simulink model "ans3"  (R2021a)
settings: Solver=VariableStepAuto  StartTime=0.0  StopTime=10.0  RelTol=1e-3
undefined symbols (not defined in the file): gcbh, xlBlockLoadCallback
libraries: xbsIndex_r4 x853, hdlBasic x20, xrbsMath_r4 x11, xrbsDSP_r4 x10, xrbsImage_r4 x4, xrbsComm_r4 x1
(part 2 of 12)

== system ans3/CIC Filter ==
  note: The CIC filter is constructed out of differentiators and integrators and
      | a sample rate change. This block provides a full precision result and is
      | dynamically built given the parameters entered in the dialog box. The
      | dynamic rebuilding script can switch which side the integrators and
      | differentiators are on and also change between an up and down sampler
      | depending on whether an Interpolator or decimator is selected respectively.
      | The number of stages selected control how many integrators and
      | differentiators are used.
  note: The Interpoiation by 48, 4 stage CIC filter occupies 116 slices.
      | The maximum clock frequency is approximately
      | 308.55 MHz in a Xilinx xc2vp2-7 part (Device speed data version:
      | PRODUCTION 1.121 2005-11-04, ISE 8.1.01i I.25 software, VHDL
      | synthesized with XST).
  In1 : Inport
  Differentiator1 : Subsystem  mask(Differentiator Stage){m=m, output_bitwidth=ceil(stages*log2(rate_change*m) + input_bitwidth), output_binpt=input_binpt}
      mask prompts: m "Differential Delay"; output_bitwidth "Output Bit Width"; output_binpt "Output Binary Point"
      mask help: Multi-Channel Differentiator
      mask init:
      | set_param(gcb, 'LinkStatus', 'none');
  Differentiator2 : Subsystem  mask(Differentiator Stage){m=m, output_bitwidth=ceil(stages*log2(rate_change*m) + input_bitwidth), output_binpt=input_binpt}
      mask prompts: m "Differential Delay"; output_bitwidth "Output Bit Width"; output_binpt "Output Binary Point"
      mask help: Multi-Channel Differentiator
      mask init:
      | set_param(gcb, 'LinkStatus', 'none');
  Differentiator3 : Subsystem  mask(Differentiator Stage){m=m, output_bitwidth=ceil(stages*log2(rate_change*m) + input_bitwidth), output_binpt=input_binpt}
      mask prompts: m "Differential Delay"; output_bitwidth "Output Bit Width"; output_binpt "Output Binary Point"
      mask help: Multi-Channel Differentiator
      mask init:
      | set_param(gcb, 'LinkStatus', 'none');
  Down Sample : hdlBasic/Down Sample  sample_ratio=rate_change  sample_phase=First Value of Frame  en=off  rst=off  latency=1  XmcBlockStatus=1  maskContainerNames=group1  block_type=dsamp  block_config=sysgen:Downsample_config
  Integrator1 : Subsystem  mask(Integrator Stage){output_bitwidth=ceil(stages*log2(rate_change*m) + input_bitwidth)}
      mask prompts: output_bitwidth "Output Bit Width"
      mask help: Multi Channel Integrator
      mask init:
      | set_param(gcb, 'LinkStatus', 'none');
      settings: CopyFcn=set_param(gcb, 'LinkStatus', 'none');
  Integrator2 : Subsystem  mask(Integrator Stage){output_bitwidth=ceil(stages*log2(rate_change*m) + input_bitwidth)}
      mask prompts: output_bitwidth "Output Bit Width"
      mask help: Multi Channel Integrator
      mask init:
      | set_param(gcb, 'LinkStatus', 'none');
      settings: CopyFcn=set_param(gcb, 'LinkStatus', 'none');
  Integrator3 : Subsystem  mask(Integrator Stage){output_bitwidth=ceil(stages*log2(rate_change*m) + input_bitwidth)}
      mask prompts: output_bitwidth "Output Bit Width"
      mask help: Multi Channel Integrator
      mask init:
      | set_param(gcb, 'LinkStatus', 'none');
      settings: CopyFcn=set_param(gcb, 'LinkStatus', 'none');
  Out1 : Outport  VectorParamsAs1DForOutWhenUnconnected=off
  wires:
  In1/1 -> Integrator1/1(In1)
  Down Sample/1 -> Differentiator1/1(In1)
  Integrator1/1(Out1) -> Integrator2/1(In1)
  Differentiator1/1(Out1) -> Differentiator2/1(In1)
  Integrator2/1(Out1) -> Integrator3/1(In1)
  Differentiator2/1(Out1) -> Differentiator3/1(In1)
  Integrator3/1(Out1) -> Down Sample/1
  Differentiator3/1(Out1) -> Out1/1

== system ans3/CIC Filter1 ==
  note: The CIC filter is constructed out of differentiators and integrators and
      | a sample rate change. This block provides a full precision result and is
      | dynamically built given the parameters entered in the dialog box. The
      | dynamic rebuilding script can switch which side the integrators and
      | differentiators are on and also change between an up and down sampler
      | depending on whether an Interpolator or decimator is selected respectively.
      | The number of stages selected control how many integrators and
      | differentiators are used.
  note: The Interpoiation by 48, 4 stage CIC filter occupies 116 slices.
      | The maximum clock frequency is approximately
      | 308.55 MHz in a Xilinx xc2vp2-7 part (Device speed data version:
      | PRODUCTION 1.121 2005-11-04, ISE 8.1.01i I.25 software, VHDL
      | synthesized with XST).
  In1 : Inport
  Differentiator1 : Subsystem  mask(Differentiator Stage){m=m, output_bitwidth=ceil(stages*log2(rate_change*m) + input_bitwidth), output_binpt=input_binpt}
      mask prompts: m "Differential Delay"; output_bitwidth "Output Bit Width"; output_binpt "Output Binary Point"
      mask help: Multi-Channel Differentiator
      mask init:
      | set_param(gcb, 'LinkStatus', 'none');
  Differentiator2 : Subsystem  mask(Differentiator Stage){m=m, output_bitwidth=ceil(stages*log2(rate_change*m) + input_bitwidth), output_binpt=input_binpt}
      mask prompts: m "Differential Delay"; output_bitwidth "Output Bit Width"; output_binpt "Output Binary Point"
      mask help: Multi-Channel Differentiator
      mask init:
      | set_param(gcb, 'LinkStatus', 'none');
  Differentiator3 : Subsystem  mask(Differentiator Stage){m=m, output_bitwidth=ceil(stages*log2(rate_change*m) + input_bitwidth), output_binpt=input_binpt}
      mask prompts: m "Differential Delay"; output_bitwidth "Output Bit Width"; output_binpt "Output Binary Point"
      mask help: Multi-Channel Differentiator
      mask init:
      | set_param(gcb, 'LinkStatus', 'none');
  Down Sample : hdlBasic/Down Sample  sample_ratio=rate_change  sample_phase=First Value of Frame  en=off  rst=off  latency=1  XmcBlockStatus=1  maskContainerNames=group1  block_type=dsamp  block_config=sysgen:Downsample_config
  Integrator1 : Subsystem  mask(Integrator Stage){output_bitwidth=ceil(stages*log2(rate_change*m) + input_bitwidth)}
      mask prompts: output_bitwidth "Output Bit Width"
      mask help: Multi Channel Integrator
      mask init:
      | set_param(gcb, 'LinkStatus', 'none');
      settings: CopyFcn=set_param(gcb, 'LinkStatus', 'none');
  Integrator2 : Subsystem  mask(Integrator Stage){output_bitwidth=ceil(stages*log2(rate_change*m) + input_bitwidth)}
      mask prompts: output_bitwidth "Output Bit Width"
      mask help: Multi Channel Integrator
      mask init:
      | set_param(gcb, 'LinkStatus', 'none');
      settings: CopyFcn=set_param(gcb, 'LinkStatus', 'none');
  Integrator3 : Subsystem  mask(Integrator Stage){output_bitwidth=ceil(stages*log2(rate_change*m) + input_bitwidth)}
      mask prompts: output_bitwidth "Output Bit Width"
      mask help: Multi Channel Integrator
      mask init:
      | set_param(gcb, 'LinkStatus', 'none');
      settings: CopyFcn=set_param(gcb, 'LinkStatus', 'none');
  Out1 : Outport  VectorParamsAs1DForOutWhenUnconnected=off
  wires:
  In1/1 -> Integrator1/1(In1)
  Down Sample/1 -> Differentiator1/1(In1)
  Integrator1/1(Out1) -> Integrator2/1(In1)
  Differentiator1/1(Out1) -> Differentiator2/1(In1)
  Integrator2/1(Out1) -> Integrator3/1(In1)
  Differentiator2/1(Out1) -> Differentiator3/1(In1)
  Integrator3/1(Out1) -> Down Sample/1
  Differentiator3/1(Out1) -> Out1/1

== system ans3/CORDIC ATAN ==
  note: The CORDIC algorithm is implemented in 3 steps.
      |
      | Step 1: Coarse Angle Rotation.  The algorithm converges only for angles between -pi/2 and pi/2, so if x < zero, the input vector is reflected
      | to the 1st or 3rd quadrant by making the x-coordinate non-negative.
      |
      | Step 2: Fine Angle Rotation.  For rectangular-to-polar conversion, the resulting vector is rotated through progressively smaller angles, such that y goes
      | to zero. In the i-th stage, the angular rotation is by either +/- atan(1/2^i), depending on whether or not its input y is less than or greater than zero.
      |
      | Step 3: Angle Correction. If there was a reflection applied in Step 1, this step applies the appropriate angle correction by subtracting it from +/- pi.
  x : Inport
  y : Inport  Port=2
  CORDIC Pipe Balance : xbsIndex_r4/Delay  rst=off  infoeditControl=Selection of Reset will increase slice count due to use of real FFs and instead of SRLs  en=off  latency=sum(pipeline)  dbl_ovrd=off  reg_retiming=off  block_type=delay
      settings: infoedit="Delay line having  configurable length.<P><P>Hardware notes: A delay line is a chain, each link of which is an SRL16 followed by a flip-flop. If register retiming is enabled, the delay line is a chain of flip-flops."  xl_area=[0, 0, 0, 0, 0, 0, 0]  block_version=VER_STRING_GOES_HERE
  CORDIC Pipe Balance1 : xbsIndex_r4/Delay  rst=off  infoeditControl=Selection of Reset will increase slice count due to use of real FFs and instead of SRLs  en=off  latency=sum(pipeline)+1  dbl_ovrd=off  reg_retiming=off  block_type=delay
      settings: infoedit="Delay line having  configurable length.<P><P>Hardware notes: A delay line is a chain, each link of which is an SRL16 followed by a flip-flop. If register retiming is enabled, the delay line is a chain of flip-flops."  xl_area=[0, 0, 0, 0, 0, 0, 0]  block_version=VER_STRING_GOES_HERE
  CORDIC Pipe Balance2 : xbsIndex_r4/Delay  rst=off  infoeditControl=Selection of Reset will increase slice count due to use of real FFs and instead of SRLs  en=off  latency=1  dbl_ovrd=off  reg_retiming=off  block_type=delay
      settings: infoedit="Delay line having  configurable length.<P><P>Hardware notes: A delay line is a chain, each link of which is an SRL16 followed by a flip-flop. If register retiming is enabled, the delay line is a chain of flip-flops."  xl_area=[0, 0, 0, 0, 0, 0, 0]  block_version=VER_STRING_GOES_HERE
  CORDIC Fine Angle PE : Subsystem  mask(CORDIC parallel PE){}
      mask init:
      | [bg,fg] = xlcmap('XBlock',0);
      | iPos = get_param(gcb,'Position');
      | iWidth=iPos(3)-iPos(1); iHeight=iPos(4)-iPos(2);
      | iCx=iWidth/2;
      | iCy=iHeight/2;
      | [logoX, logoY] = xlogo(iPos);
      mask Display:
      | patch([0 iWidth iWidth 0],[0 0 iHeight iHeight] , bg);
      | patch(logoX,logoY , fg);
      | port_label('input',1,'x');
      | port_label('input',2,'y');
      | port_label('input',3,'z');
      | port_label('output',1,'X');
      | port_label('output',2,'Z');
      | plot([0 0 iWidth iWidth 0], [0 iHeight iHeight 0 0]);
  Constant : xbsIndex_r4/Constant  const=0  gui_display_data_type=Fixed-point  arith_type=Signed (2's comp)  n_bits=pe_nbits  bin_pt=pe_binpt  preci_type=Single  exp_width=8  frac_width=24  explicit_period=off  period=1  equ=P=C  opselect=C  inp2=PCIN>>17  opr=+  inp1=P  carry=CIN  dbl_ovrd=off  block_type=constant
      settings: block_version=VER_STRING_GOES_HERE
  Quadrant Correct : Subsystem
      mask init:
      | [bg,fg] = xlcmap('XBlock',0);
      | iPos = get_param(gcb,'Position');
      | iWidth=iPos(3)-iPos(1); iHeight=iPos(4)-iPos(2);
      | iCx=iWidth/2;
      | iCy=iHeight/2;
      | [logoX, logoY] = xlogo(iPos);
      mask Display:
      | patch([0 iWidth iWidth 0],[0 0 iHeight iHeight] , bg);
      | patch(logoX,logoY , fg);
      | port_label('input',1,'Z in');
      | port_label('input',2,'sgn(y)');
      | port_label('input',3,'sgn(x)');
      | port_label('output',1,'Z');
      | plot([0 0 iWidth iWidth 0], [0 iHeight iHeight 0 0]);
  Quadrant Map : Subsystem
      mask init:
      | [bg,fg] = xlcmap('XBlock',0);
      | iPos = get_param(gcb,'Position');
      | iWidth=iPos(3)-iPos(1); iHeight=iPos(4)-iPos(2);
      | iCx=iWidth/2;
      | iCy=iHeight/2;
      | [logoX, logoY] = xlogo(iPos);
      mask Display:
      | patch([0 iWidth iWidth 0],[0 0 iHeight iHeight] , bg);
      | patch(logoX,logoY , fg);
      | port_label('input',1,'x');
      | port_label('input',2,'y');
      | port_label('output',1,'X');
      | port_label('output',2,'Y');
      | port_label('output',3,'sgn(y)');
      | port_label('output',4,'sgn(x)');
      | plot([0 0 iWidth iWidth 0], [0 iHeight iHeight 0 0]);
  X : Outport  VectorParamsAs1DForOutWhenUnconnected=off
  Z : Outport  Port=2  VectorParamsAs1DForOutWhenUnconnected=off
  wires:
  Constant/1 -> CORDIC Fine Angle PE/3(z)
  Quadrant Map/1(X) -> CORDIC Fine Angle PE/1(x)
  Quadrant Map/2(Y) -> CORDIC Fine Angle PE/2(y)
  x/1 -> Quadrant Map/1(x)
  y/1 -> Quadrant Map/2(y)
  Quadrant Map/3(sign(y)) -> CORDIC Pipe Balance/1
  Quadrant Map/4(sign(x)) -> CORDIC Pipe Balance1/1
  CORDIC Pipe Balance/1 -> Quadrant Correct/2(PI_ addsub)
  CORDIC Pipe Balance1/1 -> Quadrant Correct/3(Z MUX SEL)
  CORDIC Fine Angle PE/2(Z) -> Quadrant Correct/1(Z IN)
  Quadrant Correct/1(Z) -> Z/1
  CORDIC Fine Angle PE/1(X) -> CORDIC Pipe Balance2/1
  CORDIC Pipe Balance2/1 -> X/1

== system ans3/CORDIC DIVIDER ==
  note: The CORDIC Divider algorithm is implemented in 4 steps.
      |
      | Step 1: Co-ordinate Rotation.  The CORDIC algorithm converges only for positive values of x, so if x < zero, the input vector is
      | reflected to the 1st or 3rd quadrant by making the x-coordinate non-negative. For normalizing X and Y, Y is always mapped to
      | a non-negative value. The Divider circuit has been designed to converge for all values of X and Y, except for the most negative value .
      |
      | Step 2: Normalization.  The CORDIC algorithm converges only for y <= 2 x. For  x > y, both the inputs X and Y are shifted to the
      | left till they have a 1 in the most significant bit (MSB).  The relative shift of Y over X is recorded and passed on to the Quadrant
      | Correct Stage.
      |
      | Step 3: Linear Rotations.  For ratio calculation, the resulting vector is rotated through progressively smaller angles, such that y goes
      | to zero. In the i-th stage, the rotation yields +/- y/x, depending on whether the input y is less than or greater than zero.
      |
      | Step 4: Co-ordinate Correction. If the axis was rotated Step 1 and a relative shift was applied to Y over X, this step assigns the appropriate
      | sign to the resulting ratio and multiplies it with 2^(relative_shift of Y over X).
  x : Inport
  y : Inport  Port=2
  Constant2 : xbsIndex_r4/Constant  const=0  gui_display_data_type=Fixed-point  arith_type=Signed (2's comp)  n_bits=stages+2  bin_pt=stages  preci_type=Single  exp_width=8  frac_width=24  explicit_period=off  period=1  equ=P=C  opselect=C  inp2=PCIN>>17  opr=+  inp1=P  carry=CIN  dbl_ovrd=off  block_type=constant
      settings: block_version=VER_STRING_GOES_HERE
  Delay : xbsIndex_r4/Delay  rst=off  infoeditControl=Selection of Reset will increase slice count due to use of real FFs and instead of SRLs  en=off  latency=sum(pipeline)  dbl_ovrd=off  reg_retiming=off  block_type=delay
      settings: infoedit="Delay line having  configurable length.<P><P>Hardware notes: A delay line is a chain, each link of which is an SRL16 followed by a flip-flop. If register retiming is enabled, the delay line is a chain of flip-flops."  xl_area=[1 1 0 1 0 0 0]  block_version=VER_STRING_GOES_HERE
  Delay1 : xbsIndex_r4/Delay  rst=off  infoeditControl=Selection of Reset will increase slice count due to use of real FFs and instead of SRLs  en=off  latency=sum(pipeline)  dbl_ovrd=off  reg_retiming=off  block_type=delay
      settings: infoedit="Delay line having  configurable length.<P><P>Hardware notes: A delay line is a chain, each link of which is an SRL16 followed by a flip-flop. If register retiming is enabled, the delay line is a chain of flip-flops."  xl_area=[2 4 0 4 0 0 0]  block_version=VER_STRING_GOES_HERE
  Iterative Divider : Subsystem  mask(CORDIC Iterative Divider){}
      mask init:
      | [bg,fg] = xlcmap('XBlock',0);
      | iPos = get_param(gcb,'Position');
      | iWidth=iPos(3)-iPos(1); iHeight=iPos(4)-iPos(2);
      | iCx=iWidth/2;
      | iCy=iHeight/2;
      | [logoX, logoY] = xlogo(iPos);
      mask Display:
      | patch([0 iWidth iWidth 0],[0 0 iHeight iHeight] , bg);
      | patch(logoX,logoY , fg);
      | port_label('input',1,'x');
      | port_label('input',2,'y');
      | port_label('input',3,'z');
      | port_label('output',1,'Z');
      | plot([0 0 iWidth iWidth 0], [0 iHeight iHeight 0 0]);
  Quadrant Correct : Subsystem  mask{num_width=num_width, num_binpt=num_binpt}
      mask prompts: num_width "Data Width"; num_binpt "Data Binary Point"
      mask init:
      | [bg,fg] = xlcmap('XBlock',0);
      | iPos = get_param(gcb,'Position');
      | iWidth=iPos(3)-iPos(1); iHeight=iPos(4)-iPos(2);
      | iCx=iWidth/2;
      | iCy=iHeight/2;
      | [logoX, logoY] = xlogo(iPos);
      mask Display:
      | patch([0 iWidth iWidth 0],[0 0 iHeight iHeight] , bg);
      | patch(logoX,logoY , fg);
      | port_label('input',1,'z');
      | port_label('input',2,'sign');
      | port_label('input',3,'norm');
      | port_label('output',1,'y/x');
      | plot([0 0 iWidth iWidth 0], [0 iHeight iHeight 0 0]);
  Quadrant Map : Subsystem  mask{num_width=num_width, num_binpt=num_binpt}
      mask prompts: num_binpt "Num_bin_pt"
      mask init:
      | [bg,fg] = xlcmap('XBlock',0);
      | iPos = get_param(gcb,'Position');
      | iWidth=iPos(3)-iPos(1); iHeight=iPos(4)-iPos(2);
      | iCx=iWidth/2;
      | iCy=iHeight/2;
      | [logoX, logoY] = xlogo(iPos);
      mask Display:
      | patch([0 iWidth iWidth 0],[0 0 iHeight iHeight] , bg);
      | patch(logoX,logoY , fg);
      | port_label('input',1,'x');
      | port_label('input',2,'y');
      | port_label('output',1,'norm_x');
      | port_label('output',2,'norm_y');
      | port_label('output',3,'sign');
      | port_label('output',4,'index');
      | plot([0 0 iWidth iWidth 0], [0 iHeight iHeight 0 0]);
  div : Outport  VectorParamsAs1DForOutWhenUnconnected=off
  wires:
  Quadrant Correct/1(Z) -> div/1
  y/1 -> Quadrant Map/2(y)
  x/1 -> Quadrant Map/1(x)
  Delay1/1 -> Quadrant Correct/3(norm)
  Quadrant Map/4(index) -> Delay1/1
  Delay/1 -> Quadrant Correct/2(sign)
  Quadrant Map/3(sign) -> Delay/1
  Iterative Divider/1(Z) -> Quadrant Correct/1(z)
  Quadrant Map/2(norm_Y) -> Iterative Divider/2(y)
  Quadrant Map/1(norm_X) -> Iterative Divider/1(x)
  Constant2/1 -> Iterative Divider/3(z)

== system ans3/CORDIC LOG ==
  note: The CORDIC Natural Log algorithm is implemented in 4 steps.
      |
      | Step 1: Co-ordinate Rotation.  The CORDIC algorithm converges only for positive values of x. If x < zero, the input data is
      | converted to a non-negative number. If x = 0, a zero detect flag is passed along to the output stage. The Log circuit has been
      | designed to converge for all values of X, except for the most negative value .
      |
      | Step 2: Normalization.  The CORDIC algorithm converges only for 0.5 <= x < 1.0. During normalization, the input X is shifted to the
      | left till it has a 1 in the most significant bit.The log output is derived using the identity log( w) = 2*atanh{ (w-l) / (w+1) }.
      | Based on this identity the input w gets mapped to, X = w + 1 and Y = w - 1.
      |
      | Step 3: Hyperbolic Rotations.  For atanh{ (w-l) / (w+1) }. calculation, the resulting vector is rotated through progressively smaller
      | angles, such that y goes to zero.
      |
      | Step 4: Co-ordinate Correction. If the input was negative  a CMPLX_PI flag is porvided at the output for adding PI if a complex output is desired.
      | If a left shift was applied to X, this step adjusts the output by using the equation log (w * 2^E) = log (w) + E * log (2).
  x : Inport
  CORDIC Fine Angle PE : Subsystem  mask(CORDIC parallel PE){stages=stages, pe_nbits=pe_nbits+1, pe_binpt=pe_nbits-1, pipeline_x=pipeline, prev_stages=7, pipeline=[1  1  1  1  1  1  1]}
      mask prompts: stages "Number of Stages"; pe_nbits "Number of Bits"; pe_binpt "Binary Point Position"; pipeline_x "Pipeline Stage Value"; prev_stages "Previous Stages"; pipeline "Previous Pipeline Stage Value"
      mask init:
      | [bg,fg] = xlcmap('XBlock',0);
      | iPos = get_param(gcb,'Position');
      | iWidth=iPos(3)-iPos(1); iHeight=iPos(4)-iPos(2);
      | iCx=iWidth/2;
      | iCy=iHeight/2;
      | [logoX, logoY] = xlogo(iPos);
      | set_param(gcb,'LinkStatus', 'none');
      | sav_gcb=gcb;
      | stages = round(sum(abs(stages)));
      | if (stages == 0)
      | 	stages = prev_stages;
      | end
      | x = zeros(1,stages);
      | pipe_size = max(size(pipeline_x));
      | if pipe_size >= stages
      | 	x(1,1:stages) = pipeline_x(1,1:stages);
      | else
      | 	x(1,1:pipe_size) = pipeline_x(1,1:pipe_size);
      | end
      | 
      | if (stages ~=prev_stages)
      | 	pipeline = x;
      | 	a=find_system(sav_gcb, 'lookUnderMasks', 'all', 'FollowLinks','on','masktype', 'CORDIC iteration PE');
      | 	for i= 2:length(a)
      | 		for j=1:3
      | 		    delete_line(sav_gcb, ['CORDIC PE' int2str(i-1) '/' int2str(j)], ['CORDIC PE' int2str(i) '/' int2str(j)]);
      | 		end
      | 	end
      | 	delete_line(sav_gcb, ['CORDIC PE' int2str(length(a)) '/1'],'T1/1');
      | 	delete_line(sav_gcb, ['CORDIC PE' int2str(length(a)) '/2'],'T2/1');
      | 	delete_line(sav_gcb, ['CORDIC PE' int2str(length(a)) '/3'],'Z/1');
      | 	
      | 	for i=2:length(a)
      |       delete_block(a{i});
      | 	end
      | 	ite_stage=1;
      | 	repeat_stage=4;
      | 	dec_stage=0;
      | 	for i=2:stages
      |         ite_stage= i-dec_stage;
      | 		if(repeat_stage==ite_stage-1)
      |             ite_stage=ite_stage-1;
      | 			repeat_stage=repeat_stage*3+1;
      | 			dec_stage=dec_stage+1;
      | 		end
      |         add_block([sav_gcb '/CORDIC PE1'], [sav_gcb '/CORDIC PE' int2str(i)],'ii',int2str(ite_stage),'pipeline',['pipeline(1,' int2str(i) ')'],'position',[150+(i-1)*125, 70, 205+(i-1)*125, 130]);
      | 	end
      |     set_param([sav_gcb '/' 'T1'], 'Position', [150+stages*125, 73, 180+stages*125, 87]);
      |     set_param([sav_gcb '/' 'T2'], 'Position', [210+stages*125, 92, 225+stages*125, 108]);
      | 	set_param([sav_gcb '/' 'Z'], 'Position', [270+stages*125, 111, 270+stages*125, 129]);
      |     for i= 2:stages
      | 		for j=1:3
      | 		    add_line(sav_gcb, ['CORDIC PE' int2str(i-1) '/' int2str(j)], ['CORDIC PE' int2str(i) '/' int2str(j)]);
      | 		end
      | 	end
      |     add_line(sav_gcb, ['CORDIC PE' int2str(stages) '/1'],'T1/1');
      | 	add_line(sav_gcb, ['CORDIC PE' int2str(stages) '/2'],'T2/1');
      | 	add_line(sav_gcb, ['CORDIC PE' int2str(stages) '/3'],'Z/1');
      | 	find_system(sav_gcb, 'lookUnderMasks', 'all', 'FollowLinks', 'on', 'MaskType','Xilinx Slice Block');
      | 	set_param(sav_gcb, 'prev_stages',int2str(stages));
      | 	set_param(sav_gcb, 'pipeline', [ '[' int2str(x) ']']);
      | end
      | 
      | if (sum(pipeline~=x))
      | 	pipeline = x;
      | 	set_param(sav_gcb, 'pipeline', [ '[' int2str(x) ']']);
      | end
      mask Display:
      | patch([0 iWidth iWidth 0],[0 0 iHeight iHeight] , bg);
      | patch(logoX,logoY , fg);
      | port_label('input',1,'x');
      | port_label('input',2,'y');
      | port_label('input',3,'z');
      | port_label('input',4,'shift');
      | port_label('input',5,'sgn(x)');
      | port_label('input',6,'0_det');
      | port_label('output',1,'Z');
      | port_label('output',2,'shift');
      | port_label('output',3,'sgn(x)');
      | port_label('output',4,'0_det');
      | plot([0 0 iWidth iWidth 0], [0 iHeight iHeight 0 0]);
  Quadrant Correct : Subsystem  mask{pe_nbits=pe_nbits, pe_binpt=pe_binpt, k_val=0, k_bits=0}
      mask prompts: pe_nbits "Number of Bits"; pe_binpt "Binary Point Position"; k_val "Constant Value"; k_bits "Constant Bits"
      mask init:
      | [bg,fg] = xlcmap('XBlock',0);
      | iPos = get_param(gcb,'Position');
      | iWidth=iPos(3)-iPos(1); iHeight=iPos(4)-iPos(2);
      | iCx=iWidth/2;
      | iCy=iHeight/2;
      | [logoX, logoY] = xlogo(iPos);
      | t = pe_nbits-pe_binpt-1;
      | if (t== 0)
      | 	k_val = 0;
      | 	k_bits = 1;
      | else
      | 	k_val= t;
      | 	k_bits = ceil(log2(t+1));
      | end
      mask Display:
      | patch([0 iWidth iWidth 0],[0 0 iHeight iHeight] , bg);
      | patch(logoX,logoY , fg);
      | port_label('input',1,'X');
      | port_label('input',2,'shift');
      | port_label('input',3,'sgn(x)');
      | port_label('input',4,'0_det');
      | port_label('output',1,'log X');
      | port_label('output',2,'CMPLX_PI');
      | plot([0 0 iWidth iWidth 0], [0 iHeight iHeight 0 0]);
  Quadrant Map : Subsystem
      mask init:
      | [bg,fg] = xlcmap('XBlock',0);
      | iPos = get_param(gcb,'Position');
      | iWidth=iPos(3)-iPos(1); iHeight=iPos(4)-iPos(2);
      | iCx=iWidth/2;
      | iCy=iHeight/2;
      | [logoX, logoY] = xlogo(iPos);
      mask Display:
      | patch([0 iWidth iWidth 0],[0 0 iHeight iHeight] , bg);
      | patch(logoX,logoY , fg);
      | port_label('input',1,'x');
      | port_label('output',1,'X');
      | port_label('output',2,'Y');
      | port_label('output',3,'Z');
      | port_label('output',4,'shift');
      | port_label('output',5,'sgn(x)');
      | port_label('output',6,'0_det');
      | plot([0 0 iWidth iWidth 0], [0 iHeight iHeight 0 0]);
  logx : Outport  VectorParamsAs1DForOutWhenUnconnected=off
  CMPLX_PI : Outport  Port=2  VectorParamsAs1DForOutWhenUnconnected=off
  wires:
  CORDIC Fine Angle PE/3(sign_dly) -> Quadrant Correct/3(sign_x)
  CORDIC Fine Angle PE/2(shift_dly) -> Quadrant Correct/2(shift)
  Quadrant Map/5(sign) -> CORDIC Fine Angle PE/5(sign)
  Quadrant Map/6(zero_detect) -> CORDIC Fine Angle PE/6(zero_detect)
  Quadrant Map/4(shift1) -> CORDIC Fine Angle PE/4(shift1)
  Quadrant Map/3(shift) -> CORDIC Fine Angle PE/3(z)
  Quadrant Map/2(Y) -> CORDIC Fine Angle PE/2(y)
  Quadrant Map/1(X) -> CORDIC Fine Angle PE/1(x)
  Quadrant Correct/2(CMPLX_PI) -> CMPLX_PI/1
  CORDIC Fine Angle PE/4(zero_detect_dly) -> Quadrant Correct/4(zero_detect)
  x/1 -> Quadrant Map/1(x)
  CORDIC Fine Angle PE/1(Z) -> Quadrant Correct/1(X)
  Quadrant Correct/1(Z) -> logx/1

== system ans3/CORDIC SINCOS ==
  note: The CORDIC algorithm is implemented in 3 steps.
      |
      | Step 1: Coarse Angle Rotation.  The algorithm converges only for angles between -pi/2 and pi/2. If  z > pi/2, the input angle is reflected
      |  to the 1st quadrant by subtracting pi/2 from the input angle. When z < -pi/2, the input angle is reflected back to the 3rd quadrant by adding
      | pi/2 to the input angle .
      |
      | Step 2: Fine Angle Rotation.  By setting x equal to 1/1.646760 and y equal to 0, the rotational mode CORDIC processor yields cosine and sine
      | of the input angle Z.
      |
      | Step 3: Angle Correction. If there was a reflection applied in Step 1, this step applies the appropriate correction .
  z : Inport
  CORDIC Fine Angle PE : Subsystem  mask(CORDIC parallel PE){}
      mask init:
      | [bg,fg] = xlcmap('XBlock',0);
      | iPos = get_param(gcb,'Position');
      | iWidth=iPos(3)-iPos(1); iHeight=iPos(4)-iPos(2);
      | iCx=iWidth/2;
      | iCy=iHeight/2;
      | [logoX, logoY] = xlogo(iPos);
      mask Display:
      | patch([0 iWidth iWidth 0],[0 0 iHeight iHeight] , bg);
      | patch(logoX,logoY , fg);
      | port_label('input',1,'x');
      | port_label('input',2,'y');
      | port_label('input',3,'z');
      | port_label('output',1,'X');
      | port_label('output',2,'Y');
      | plot([0 0 iWidth iWidth 0], [0 iHeight iHeight 0 0]);
  Constant : xbsIndex_r4/Constant  const=1/1.646760  gui_display_data_type=Fixed-point  arith_type=Signed (2's comp)  n_bits=pe_nbits  bin_pt=pe_binpt  preci_type=Single  exp_width=8  frac_width=24  explicit_period=off  period=1  equ=P=C  opselect=C  inp2=PCIN>>17  opr=+  inp1=P  carry=CIN  dbl_ovrd=off  block_type=constant
      settings: block_version=VER_STRING_GOES_HERE
  Constant1 : xbsIndex_r4/Constant  const=0  gui_display_data_type=Fixed-point  arith_type=Signed (2's comp)  n_bits=pe_nbits  bin_pt=pe_binpt  preci_type=Single  exp_width=8  frac_width=24  explicit_period=off  period=1  equ=P=C  opselect=C  inp2=PCIN>>17  opr=+  inp1=P  carry=CIN  dbl_ovrd=off  block_type=constant
      settings: block_version=VER_STRING_GOES_HERE
  Delay1 : xbsIndex_r4/Delay  rst=off  infoeditControl=Selection of Reset will increase slice count due to use of real FFs and instead of SRLs  en=off  latency=sum(pipeline)+2  dbl_ovrd=off  reg_retiming=off  block_type=delay
      settings: infoedit="Delay line having  configurable length.<P><P>Hardware notes: A delay line is a chain, each link of which is an SRL16 followed by a flip-flop. If register retiming is enabled, the delay line is a chain of flip-flops."  xl_area=[1 1 0 1 0 0 0]  block_version=VER_STRING_GOES_HERE
  Delay4 : xbsIndex_r4/Delay  rst=off  infoeditControl=Selection of Reset will increase slice count due to use of real FFs and instead of SRLs  en=off  latency=sum(pipeline)+1  dbl_ovrd=off  reg_retiming=off  block_type=delay
      settings: infoedit="Delay line having  configurable length.<P><P>Hardware notes: A delay line is a chain, each link of which is an SRL16 followed by a flip-flop. If register retiming is enabled, the delay line is a chain of flip-flops."  xl_area=[1 1 0 1 0 0 0]  block_version=VER_STRING_GOES_HERE
  Quadrant Correct : Subsystem
      mask init:
      | [bg,fg] = xlcmap('XBlock',0);
      | iPos = get_param(gcb,'Position');
      | iWidth=iPos(3)-iPos(1); iHeight=iPos(4)-iPos(2);
      | iCx=iWidth/2;
      | iCy=iHeight/2;
      | [logoX, logoY] = xlogo(iPos);
      mask Display:
      | patch([0 iWidth iWidth 0],[0 0 iHeight iHeight] , bg);
      | patch(logoX,logoY , fg);
      | port_label('input',1,'x');
      | port_label('input',2,'y');
      | port_label('input',3,'angle_map');
      | port_label('input',4,'sgn(z)');
      | port_label('output',1,'cos');
      | port_label('output',2,'sin');
      | plot([0 0 iWidth iWidth 0], [0 iHeight iHeight 0 0]);
  Quadrant Map : Subsystem
      mask init:
      | [bg,fg] = xlcmap('XBlock',0);
      | iPos = get_param(gcb,'Position');
      | iWidth=iPos(3)-iPos(1); iHeight=iPos(4)-iPos(2);
      | iCx=iWidth/2;
      | iCy=iHeight/2;
      | [logoX, logoY] = xlogo(iPos);
      mask Display:
      | patch([0 iWidth iWidth 0],[0 0 iHeight iHeight] , bg);
      | patch(logoX,logoY , fg);
      | port_label('input',1,'z');
      | port_label('output',1,'z');
      | port_label('output',2,'angle_map');
      | port_label('output',3,'sgn(z)');
      | plot([0 0 iWidth iWidth 0], [0 iHeight iHeight 0 0]);
  cos : Outport  VectorParamsAs1DForOutWhenUnconnected=off
  sin : Outport  Port=2  VectorParamsAs1DForOutWhenUnconnected=off
  wires:
  CORDIC Fine Angle PE/1(X) -> Quadrant Correct/1(cos)
  CORDIC Fine Angle PE/2(Y) -> Quadrant Correct/2(sin)
  Delay1/1 -> Quadrant Correct/4(sgn(z))
  Delay4/1 -> Quadrant Correct/3(angle_map)
  z/1 -> Quadrant Map/1(z)
  Quadrant Map/2(angle_map) -> Delay4/1
  Quadrant Map/3(sgn_z) -> Delay1/1
  Quadrant Map/1(Z) -> CORDIC Fine Angle PE/3(z)
  Constant/1 -> CORDIC Fine Angle PE/1(x)
  Constant1/1 -> CORDIC Fine Angle PE/2(y)
  Quadrant Correct/2(sine) -> sin/1
  Quadrant Correct/1(cosine) -> cos/1

== system ans3/CORDIC SQRT ==
  note: The CORDIC Square Root algorithm is implemented in 4 steps.
      |
      | Step 1: Co-ordinate Rotation.  The CORDIC algorithm converges only for positive values of x. If x < zero, the input data is
      | converted to a non-negative number. If x = 0, a zero detect flag is passed along. The Square Root circuit has been designed to
      | converge for all values of X, except for the most negative value .
      |
      | Step 2: Normalization.  The CORDIC algorithm converges only for 0.25 <= x < 1.0. During normalization, the input X is shifted to the
      | left till it has a 1 in the most significant bit after the signed bit. If the left shift resullted in an odd number of shift values, a right shift is
      | performed resulting in an even number of left shifts. The shift value is divided by 2 and passed on to the quadrant correct stage. The
      | square root is derived using the identity sqrt( w) = sqrt{ (w + 1/4)^2 - (w - 1/4)^2). Based on this identity the input w gets mapped to,
      | X = w + 0.25 and Y = w - 0.25.
      |
      | Step 3: Hyperbolic Rotations.  For sqrt(x^2 - y^2) calculation, the resulting vector is rotated through progressively smaller angles, such
      | that y goes to zero.
      |
      | Step 4: Co-ordinate Correction. If the input was negative and a left shift was applied to X, this step assigns the appropriate
      | sign to the resulting ratio and multiplies it with 2^(-shift). If the input was zero, the zero detect flag is used to set the output
      | to 0.
  x : Inport
  CORDIC Fine Angle PE : Subsystem  mask(CORDIC parallel PE){stages=stages, pe_nbits=norm_nbits+1, pe_binpt=norm_binpt, pipeline_x=pipeline, prev_stages=11, pipeline=[1  1  1  1  1  1  1  1  1  1  1]}
      mask prompts: stages "Number of Stages"; pe_nbits "Number of Bits"; pe_binpt "Binary Point Position"; pipeline_x "Pipeline Stage Value"; prev_stages "Previous Stages"; pipeline "Previous Pipeline Stage Value"
      mask init:
      | [bg,fg] = xlcmap('XBlock',0);
      | iPos = get_param(gcb,'Position');
      | iWidth=iPos(3)-iPos(1); iHeight=iPos(4)-iPos(2);
      | iCx=iWidth/2;
      | iCy=iHeight/2;
      | [logoX, logoY] = xlogo(iPos);
      | set_param(gcb,'LinkStatus', 'none');
      | sav_gcb=gcb;
      | stages = round(sum(abs(stages)));
      | if (stages == 0)
      | 	stages = prev_stages;
      | end
      | x = zeros(1,stages);
      | pipe_size = max(size(pipeline_x));
      | if pipe_size >= stages
      | 	x(1,1:stages) = pipeline_x(1,1:stages);
      | else
      | 	x(1,1:pipe_size) = pipeline_x(1,1:pipe_size);
      | end
      | 
      | if (stages ~=prev_stages)
      | 	pipeline = x;
      | 	a=find_system(sav_gcb, 'lookUnderMasks', 'all', 'FollowLinks','on','masktype', 'CORDIC iteration PE');
      | 	for i= 2:length(a)
      | 		for j=1:2
      | 		    delete_line(sav_gcb, ['CORDIC PE' int2str(i-1) '/' int2str(j)], ['CORDIC PE' int2str(i) '/' int2str(j)]);
      | 		end
      | 	end
      | 	delete_line(sav_gcb, ['CORDIC PE' int2str(length(a)) '/1'],'X/1');
      | 	delete_line(sav_gcb, ['CORDIC PE' int2str(length(a)) '/2'],'Terminator/1');
      | 	
      | 	for i=2:length(a)
      |       delete_block(a{i});
      | 	end
      | 	ite_stage=1;
      | 	repeat_stage=4;
      | 	dec_stage=0;
      | 	for i=2:stages
      |         ite_stage= i-dec_stage;
      | 		if(repeat_stage==ite_stage-1)
      |             ite_stage=ite_stage-1;
      | 			repeat_stage=repeat_stage*3+1;
      | 			dec_stage=dec_stage+1;
      | 		end
      |         add_block([sav_gcb '/CORDIC PE1'], [sav_gcb '/CORDIC PE' int2str(i)],'ii',int2str(ite_stage),'pipeline',['pipeline(1,' int2str(i) ')'],'position',[150+(i-1)*125, 70, 205+(i-1)*125, 130]);
      | 	end
      |     set_param([sav_gcb '/' 'X'], 'Position', [150+stages*125, 78, 180+stages*125, 92]);
      |     set_param([sav_gcb '/' 'Terminator'], 'Position', [210+stages*125, 107, 225+stages*125, 123]);
      |     for i= 2:stages
      | 		for j=1:2
      | 		    add_line(sav_gcb, ['CORDIC PE' int2str(i-1) '/' int2str(j)], ['CORDIC PE' int2str(i) '/' int2str(j)]);
      | 		end
      | 	end
      |     add_line(sav_gcb, ['CORDIC PE' int2str(stages) '/1'],'X/1');
      | 	add_line(sav_gcb, ['CORDIC PE' int2str(stages) '/2'],'Terminator/1');
      | 	find_system(sav_gcb, 'lookUnderMasks', 'all', 'FollowLinks', 'on', 'MaskType','Xilinx Slice Block');
      | 	set_param(sav_gcb, 'prev_stages',int2str(stages));
      | 	set_param(sav_gcb, 'pipeline', [ '[' int2str(x) ']']);
      | end
      | 
      | if (sum(pipeline~=x))
      | 	pipeline = x;
      | 	set_param(sav_gcb, 'pipeline', [ '[' int2str(x) ']']);
      | end
      mask Display:
      | patch([0 iWidth iWidth 0],[0 0 iHeight iHeight] , bg);
      | patch(logoX,logoY , fg);
      | port_label('input',1,'x');
      | port_label('input',2,'y');
      | port_label('input',3,'sgn(x)');
      | port_label('input',4,'shift');
      | port_label('input',5,'0_det');
      | port_label('output',1,'X');
      | port_label('output',2,'sgn(x)');
      | port_label('output',3,'shift');
      | port_label('output',4,'0_det');
      | plot([0 0 iWidth iWidth 0], [0 iHeight iHeight 0 0]);
  Quadrant Correct : Subsystem
      mask init:
      | [bg,fg] = xlcmap('XBlock',0);
      | iPos = get_param(gcb,'Position');
      | iWidth=iPos(3)-iPos(1); iHeight=iPos(4)-iPos(2);
      | iCx=iWidth/2;
      | iCy=iHeight/2;
      | [logoX, logoY] = xlogo(iPos);
      mask Display:
      | patch([0 iWidth iWidth 0],[0 0 iHeight iHeight] , bg);
      | patch(logoX,logoY , fg);
      | port_label('input',1,'X');
      | port_label('input',2,'sgn(x)');
      | port_label('input',3,'shift');
      | port_label('input',4,'0_det');
      | port_label('output',1,'X');
      | plot([0 0 iWidth iWidth 0], [0 iHeight iHeight 0 0]);
  Quadrant Map : Subsystem
      mask init:
      | [bg,fg] = xlcmap('XBlock',0);
      | iPos = get_param(gcb,'Position');
      | iWidth=iPos(3)-iPos(1); iHeight=iPos(4)-iPos(2);
      | iCx=iWidth/2;
      | iCy=iHeight/2;
      | [logoX, logoY] = xlogo(iPos);
      mask Display:
      | patch([0 iWidth iWidth 0],[0 0 iHeight iHeight] , bg);
      | patch(logoX,logoY , fg);
      | port_label('input',1,'x');
      | port_label('output',1,'X');
      | port_label('output',2,'Y');
      | port_label('output',3,'sgn(x)');
      | port_label('output',4,'shift');
      | port_label('output',5,'0_det');
      | plot([0 0 iWidth iWidth 0], [0 iHeight iHeight 0 0]);
  X : Outport  VectorParamsAs1DForOutWhenUnconnected=off
  wires:
  CORDIC Fine Angle PE/4(zero_detect_dly) -> Quadrant Correct/4(zero_detect)
  Quadrant Map/5(zero_detect) -> CORDIC Fine Angle PE/5(zero_detect)
  CORDIC Fine Angle PE/3(shift_dly) -> Quadrant Correct/3(shift)
  CORDIC Fine Angle PE/2(sign_dly) -> Quadrant Correct/2(sign_x)
  Quadrant Map/4(shift) -> CORDIC Fine Angle PE/4(shift)
  Quadrant Map/3(sign(x)) -> CORDIC Fine Angle PE/3(sign)
  x/1 -> Quadrant Map/1(x)
  CORDIC Fine Angle PE/1(X) -> Quadrant Correct/1(X)
  Quadrant Correct/1(Z) -> X/1
  Quadrant Map/2(Y) -> CORDIC Fine Angle PE/2(y)
  Quadrant Map/1(X) -> CORDIC Fine Angle PE/1(x)

== system ans3/Reset Generator ==
  rst : Inport
  Clock Enable Probe : xbsIndex_r4/Clock Enable Probe  inherit_constraints=on  block_type=ceprobe
      settings: infoedit="Clock enable extractor.  Produces a Boolean output that mirrors the hardware clock enable associated with the input sample rate.<br><br>Hardware notes: in hardware this block costs nothing."
  Constant : xbsIndex_r4/Constant  const=1.0  gui_display_data_type=Fixed-point  arith_type=Boolean  n_bits=1  bin_pt=0  preci_type=Single  exp_width=8  frac_width=24  explicit_period=off  period=1  equ=P=C  opselect=C  inp2=PCIN>>17  opr=+  inp1=P  carry=CIN  dbl_ovrd=off  block_type=constant
  Down Sample : xbsIndex_r4/Down Sample  sample_ratio=5  sample_phase="Last Value of Frame  (most efficient)"  en=off  rst=off  latency=1  dbl_ovrd=off  block_type=dsamp
  Down Sample1 : xbsIndex_r4/Down Sample  sample_ratio=2  sample_phase="Last Value of Frame  (most efficient)"  en=off  rst=off  latency=3  dbl_ovrd=off  block_type=dsamp
  Inverter : xbsIndex_r4/Inverter  en=off  latency=1  dbl_ovrd=off  block_type=inv
  Inverter1 : xbsIndex_r4/Inverter  en=off  latency=1  dbl_ovrd=off  block_type=inv
  Logical : xbsIndex_r4/Logical  logical_function=AND  inputs=2  en=off  latency=1  precision=Full  arith_type=Unsigned  n_bits=16  bin_pt=0  align_bp=on  dbl_ovrd=off  block_type=logical
  Logical1 : xbsIndex_r4/Logical  logical_function=OR  inputs=2  en=off  latency=1  precision=Full  arith_type=Unsigned  n_bits=16  bin_pt=0  align_bp=on  dbl_ovrd=off  block_type=logical
  Register : xbsIndex_r4/Register  init=0  rst=on  en=on  dbl_ovrd=off  block_type=register
  rst5 : Outport  VectorParamsAs1DForOutWhenUnconnected=off
  rst2 : Outport  Port=2  VectorParamsAs1DForOutWhenUnconnected=off
  rdy : Outport  Port=3  VectorParamsAs1DForOutWhenUnconnected=off
  wires:
  Down Sample/1 -> Clock Enable Probe/1, Logical1/1, rst5/1  "slow_rst"
  rst/1 -> Inverter/1, Register/3
  Clock Enable Probe/1 -> Logical/1
  Inverter/1 -> Logical/2
  Constant/1 -> Register/1
  Logical/1 -> Register/2
  Register/1 -> Down Sample/1, Logical1/2, Down Sample1/1  "reg_out"
  Logical1/1 -> Inverter1/1
  Down Sample1/1 -> rst2/1
  Inverter1/1 -> rdy/1  "rdy_out"

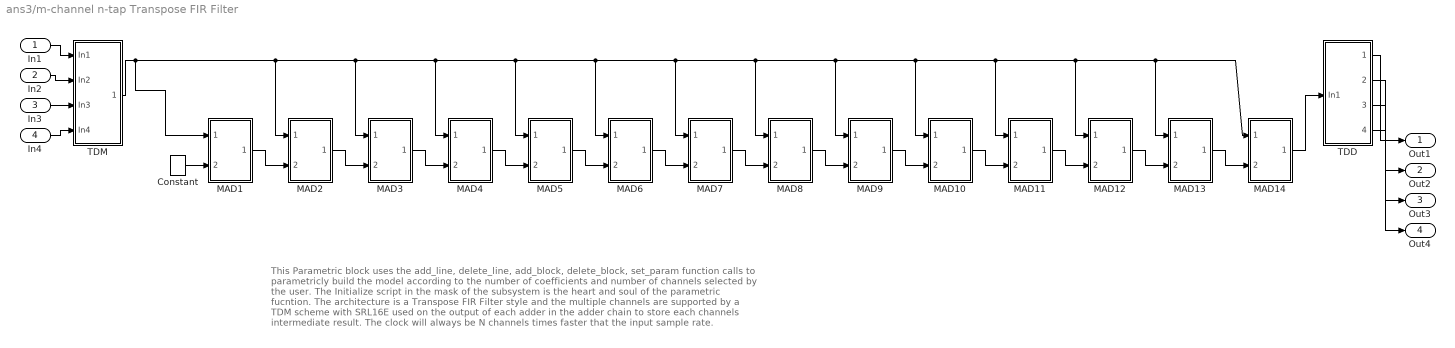
== system ans3/m-channel n-tap Transpose FIR Filter ==
  note: This Parametric block uses the add_line, delete_line, add_block, delete_block, set_param function calls to parametricly
      | build the model according to the number of coefficients and number of channels selected by the user. The Initialize script in
      | the mask of the subsystem is the heart and soul of the parametric fucntion.
      |
      | The architecture is a Transpose FIR Filter style and the multiple channels are supported by a TDM scheme with SRL16E used
      | on the output of each adder in the adder chain to store each channels intermediate result. The clock will always be N channels
      | times faster that the input sample rate.
  In1 : Inport
  In2 : Inport  Port=2
  In3 : Inport  Port=3
  In4 : Inport  Port=4
  Constant : xbsIndex_r4/Constant  const=0  gui_display_data_type=Fixed-point  arith_type=Unsigned  n_bits=1  bin_pt=0  preci_type=Single  exp_width=8  frac_width=24  explicit_period=off  period=1  equ=P=C  opselect=C  inp2=PCIN>>17  opr=+  inp1=P  carry=CIN  dbl_ovrd=off  block_type=constant
      settings: block_version=VER_STRING_GOES_HERE
  MAD1 : Subsystem  mask(MAD Block){coef=coef_array(1), coef_bitwidth=coef_bitwidth, coef_binpt=coef_binpt, channels=channels}
      mask prompts: coef "Coefficient Value"; coef_bitwidth "Coefficient Bit Width"; coef_binpt "Coefficient Binary Point"; channels "Number of Channels"
  MAD10 : Subsystem  mask(MAD Block){coef=coef_array(10), coef_bitwidth=coef_bitwidth, coef_binpt=coef_binpt, channels=channels}
      mask prompts: coef "Coefficient Value"; coef_bitwidth "Coefficient Bit Width"; coef_binpt "Coefficient Binary Point"; channels "Number of Channels"
  MAD11 : Subsystem  mask(MAD Block){coef=coef_array(11), coef_bitwidth=coef_bitwidth, coef_binpt=coef_binpt, channels=channels}
      mask prompts: coef "Coefficient Value"; coef_bitwidth "Coefficient Bit Width"; coef_binpt "Coefficient Binary Point"; channels "Number of Channels"
  MAD12 : Subsystem  mask(MAD Block){coef=coef_array(12), coef_bitwidth=coef_bitwidth, coef_binpt=coef_binpt, channels=channels}
      mask prompts: coef "Coefficient Value"; coef_bitwidth "Coefficient Bit Width"; coef_binpt "Coefficient Binary Point"; channels "Number of Channels"
  MAD13 : Subsystem  mask(MAD Block){coef=coef_array(13), coef_bitwidth=coef_bitwidth, coef_binpt=coef_binpt, channels=channels}
      mask prompts: coef "Coefficient Value"; coef_bitwidth "Coefficient Bit Width"; coef_binpt "Coefficient Binary Point"; channels "Number of Channels"
  MAD14 : Subsystem  mask(MAD Block){coef=coef_array(14), coef_bitwidth=coef_bitwidth, coef_binpt=coef_binpt, channels=channels}
      mask prompts: coef "Coefficient Value"; coef_bitwidth "Coefficient Bit Width"; coef_binpt "Coefficient Binary Point"; channels "Number of Channels"
  MAD2 : Subsystem  mask(MAD Block){coef=coef_array(2), coef_bitwidth=coef_bitwidth, coef_binpt=coef_binpt, channels=channels}
      mask prompts: coef "Coefficient Value"; coef_bitwidth "Coefficient Bit Width"; coef_binpt "Coefficient Binary Point"; channels "Number of Channels"
  MAD3 : Subsystem  mask(MAD Block){coef=coef_array(3), coef_bitwidth=coef_bitwidth, coef_binpt=coef_binpt, channels=channels}
      mask prompts: coef "Coefficient Value"; coef_bitwidth "Coefficient Bit Width"; coef_binpt "Coefficient Binary Point"; channels "Number of Channels"
  MAD4 : Subsystem  mask(MAD Block){coef=coef_array(4), coef_bitwidth=coef_bitwidth, coef_binpt=coef_binpt, channels=channels}
      mask prompts: coef "Coefficient Value"; coef_bitwidth "Coefficient Bit Width"; coef_binpt "Coefficient Binary Point"; channels "Number of Channels"
  MAD5 : Subsystem  mask(MAD Block){coef=coef_array(5), coef_bitwidth=coef_bitwidth, coef_binpt=coef_binpt, channels=channels}
      mask prompts: coef "Coefficient Value"; coef_bitwidth "Coefficient Bit Width"; coef_binpt "Coefficient Binary Point"; channels "Number of Channels"
  MAD6 : Subsystem  mask(MAD Block){coef=coef_array(6), coef_bitwidth=coef_bitwidth, coef_binpt=coef_binpt, channels=channels}
      mask prompts: coef "Coefficient Value"; coef_bitwidth "Coefficient Bit Width"; coef_binpt "Coefficient Binary Point"; channels "Number of Channels"
  MAD7 : Subsystem  mask(MAD Block){coef=coef_array(7), coef_bitwidth=coef_bitwidth, coef_binpt=coef_binpt, channels=channels}
      mask prompts: coef "Coefficient Value"; coef_bitwidth "Coefficient Bit Width"; coef_binpt "Coefficient Binary Point"; channels "Number of Channels"
  MAD8 : Subsystem  mask(MAD Block){coef=coef_array(8), coef_bitwidth=coef_bitwidth, coef_binpt=coef_binpt, channels=channels}
      mask prompts: coef "Coefficient Value"; coef_bitwidth "Coefficient Bit Width"; coef_binpt "Coefficient Binary Point"; channels "Number of Channels"
  MAD9 : Subsystem  mask(MAD Block){coef=coef_array(9), coef_bitwidth=coef_bitwidth, coef_binpt=coef_binpt, channels=channels}
      mask prompts: coef "Coefficient Value"; coef_bitwidth "Coefficient Bit Width"; coef_binpt "Coefficient Binary Point"; channels "Number of Channels"
  TDD : Subsystem  mask(TDD){}
      mask help: Multi-Channel Time Division DeMultiplexer
  TDM : Subsystem
  Out1 : Outport  VectorParamsAs1DForOutWhenUnconnected=off
  Out2 : Outport  Port=2  VectorParamsAs1DForOutWhenUnconnected=off
  Out3 : Outport  Port=3  VectorParamsAs1DForOutWhenUnconnected=off
  Out4 : Outport  Port=4  VectorParamsAs1DForOutWhenUnconnected=off
  wires:
  TDD/4(Out4) -> Out4/1
  TDD/3(Out3) -> Out3/1
  TDD/2(Out2) -> Out2/1
  In4/1 -> TDM/4(In4)
  In3/1 -> TDM/3(In3)
  In2/1 -> TDM/2(In2)
  TDD/1(Out1) -> Out1/1
  In1/1 -> TDM/1(In1)
  Constant/1 -> MAD1/2(In2)
  TDM/1(Out1) -> MAD13/1(In1), MAD14/1(In1), MAD12/1(In1), MAD11/1(In1), MAD10/1(In1), MAD9/1(In1), MAD8/1(In1), MAD7/1(In1), MAD6/1(In1), MAD5/1(In1), MAD4/1(In1), MAD3/1(In1), MAD2/1(In1), MAD1/1(In1)
  MAD1/1(Out1) -> MAD2/2(In2)
  MAD2/1(Out1) -> MAD3/2(In2)
  MAD3/1(Out1) -> MAD4/2(In2)
  MAD4/1(Out1) -> MAD5/2(In2)
  MAD5/1(Out1) -> MAD6/2(In2)
  MAD6/1(Out1) -> MAD7/2(In2)
  MAD7/1(Out1) -> MAD8/2(In2)
  MAD8/1(Out1) -> MAD9/2(In2)
  MAD9/1(Out1) -> MAD10/2(In2)
  MAD10/1(Out1) -> MAD11/2(In2)
  MAD11/1(Out1) -> MAD12/2(In2)
  MAD12/1(Out1) -> MAD13/2(In2)
  MAD13/1(Out1) -> MAD14/2(In2)
  MAD14/1(Out1) -> TDD/1(In1)

== system ans3/CIC Filter/Differentiator1 ==
  In1 : Inport
  AddSub : hdlBasic/AddSub  mode=Subtraction  use_carryin=off  use_carryout=off  en=off  latency=1  precision=User Defined  arith_type="Signed  (2's comp)"  n_bits=output_bitwidth  bin_pt=output_binpt  quantization=Truncate  overflow=Wrap  use_behavioral_HDL=on  hw_selection=Fabric  pipelined=off  use_rpm=on  XmcBlockStatus=1  maskContainerNames=tabcontainer1  block_type=addsub  block_config=sysgen:Addsub_config
  Delay : hdlBasic/Delay  rst=off  en=off  latency=m  reg_retiming=off  XmcBlockStatus=1  maskContainerNames=group1  block_type=delay  block_config=sysgen:Delay_config
  Out1 : Outport  VectorParamsAs1DForOutWhenUnconnected=off
  wires:
  In1/1 -> Delay/1, AddSub/1
  AddSub/1 -> Out1/1
  Delay/1 -> AddSub/2

== system ans3/CIC Filter/Differentiator2 ==
  In1 : Inport
  AddSub : hdlBasic/AddSub  mode=Subtraction  use_carryin=off  use_carryout=off  en=off  latency=1  precision=User Defined  arith_type="Signed  (2's comp)"  n_bits=output_bitwidth  bin_pt=output_binpt  quantization=Truncate  overflow=Wrap  use_behavioral_HDL=on  hw_selection=Fabric  pipelined=off  use_rpm=on  XmcBlockStatus=1  maskContainerNames=tabcontainer1  block_type=addsub  block_config=sysgen:Addsub_config
  Delay : hdlBasic/Delay  rst=off  en=off  latency=m  reg_retiming=off  XmcBlockStatus=1  maskContainerNames=group1  block_type=delay  block_config=sysgen:Delay_config
  Out1 : Outport  VectorParamsAs1DForOutWhenUnconnected=off
  wires:
  Delay/1 -> AddSub/2
  AddSub/1 -> Out1/1
  In1/1 -> AddSub/1, Delay/1

== system ans3/CIC Filter/Differentiator3 ==
  In1 : Inport
  AddSub : hdlBasic/AddSub  mode=Subtraction  use_carryin=off  use_carryout=off  en=off  latency=1  precision=User Defined  arith_type="Signed  (2's comp)"  n_bits=output_bitwidth  bin_pt=output_binpt  quantization=Truncate  overflow=Wrap  use_behavioral_HDL=on  hw_selection=Fabric  pipelined=off  use_rpm=on  XmcBlockStatus=1  maskContainerNames=tabcontainer1  block_type=addsub  block_config=sysgen:Addsub_config
  Delay : hdlBasic/Delay  rst=off  en=off  latency=m  reg_retiming=off  XmcBlockStatus=1  maskContainerNames=group1  block_type=delay  block_config=sysgen:Delay_config
  Out1 : Outport  VectorParamsAs1DForOutWhenUnconnected=off
  wires:
  Delay/1 -> AddSub/2
  AddSub/1 -> Out1/1
  In1/1 -> AddSub/1, Delay/1

== system ans3/CIC Filter/Integrator1 ==
  In1 : Inport
  Accumulator : hdlBasic/Accumulator  operation=Add  n_bits=output_bitwidth  overflow=Wrap  scale=1  rst=off  hasbypass=off  en=off  latency=1  msb_inp=100  msb=100  lsb=-100  use_behavioral_HDL=on  implementation=Fabric  XmcBlockStatus=1  maskContainerNames=group3  block_type=accum  block_config=sysgen:Accum_config  block_width=566  block_height=845
  Out1 : Outport  VectorParamsAs1DForOutWhenUnconnected=off
  wires:
  In1/1 -> Accumulator/1
  Accumulator/1 -> Out1/1
